simulink model "untitled"  (R2023b)
settings: Solver=VariableStepAuto  StartTime=0.0  StopTime=10.0  RelTol=1e-3
settings Model: Creator=alberto  LastModifiedBy=alberto

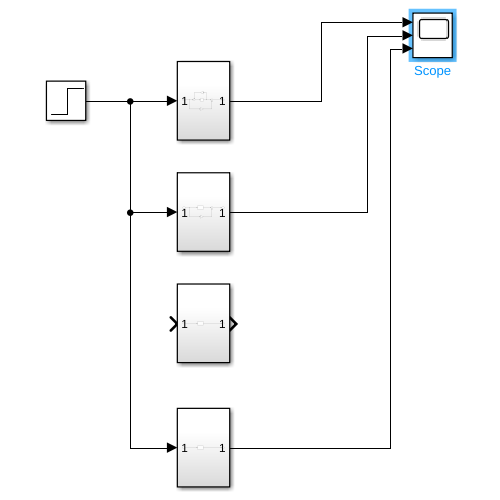
[thumbnail: Simulink's stored preview of the top-level diagram]
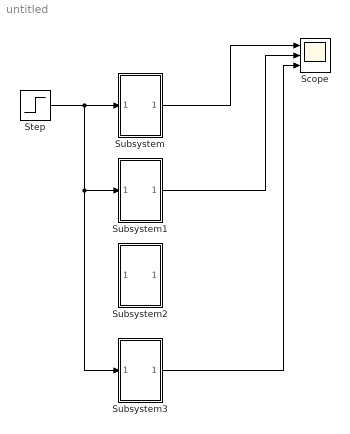
== system untitled ==
  Scope : Scope  NumInputPorts=3
  Step : Step  SampleTime=0
  Subsystem : Subsystem
  Subsystem1 : Subsystem
  Subsystem2 : Subsystem
  Subsystem3 : Subsystem
  wires:
  Subsystem/1(Out1) -> Scope/1
  Step/1 -> Subsystem3/1(In1), Subsystem1/1(In1), Subsystem/1(In1)
  Subsystem1/1(Out1) -> Scope/2
  Subsystem3/1(Out1) -> Scope/3

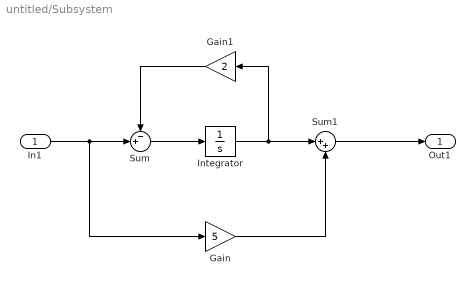
== system untitled/Subsystem ==
  In1 : Inport
  Gain : Gain  Gain=5
  Gain1 : Gain  Gain=2
  Integrator : Integrator
  Sum : Sum  Inputs=-+|
  Sum1 : Sum  Inputs=|++
  Out1 : Outport
  wires:
  Sum/1 -> Integrator/1
  Gain/1 -> Sum1/2
  Sum1/1 -> Out1/1
  Integrator/1 -> Sum1/1, Gain1/1
  In1/1 -> Sum/2, Gain/1
  Gain1/1 -> Sum/1

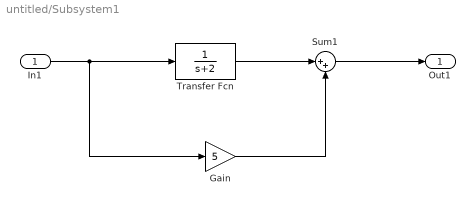
== system untitled/Subsystem1 ==
  In1 : Inport
  Gain : Gain  Gain=5
  Sum1 : Sum  Inputs=|++
  Transfer Fcn : TransferFcn  Denominator=[1 2]
  Out1 : Outport
  wires:
  In1/1 -> Transfer Fcn/1, Gain/1
  Sum1/1 -> Out1/1
  Gain/1 -> Sum1/2
  Transfer Fcn/1 -> Sum1/1

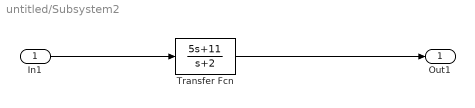
== system untitled/Subsystem2 ==
  In1 : Inport
  Transfer Fcn : TransferFcn  Numerator=[5 11]  Denominator=[1 2]
  Out1 : Outport
  wires:
  In1/1 -> Transfer Fcn/1
  Transfer Fcn/1 -> Out1/1

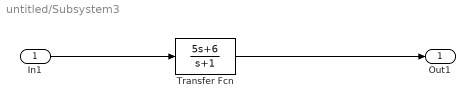
== system untitled/Subsystem3 ==
  In1 : Inport
  Transfer Fcn : TransferFcn  Numerator=[5 6]  Denominator=[1 1]
  Out1 : Outport
  wires:
  Transfer Fcn/1 -> Out1/1
  In1/1 -> Transfer Fcn/1
